simulink subsystem "DataLoader_Single_Array"  (R2019b)
settings: Solver=VariableStepAuto  StartTime=0.0  StopTime=10.0  RelTol=1e-3
settings Model: Creator=toons  LastModifiedBy=toons

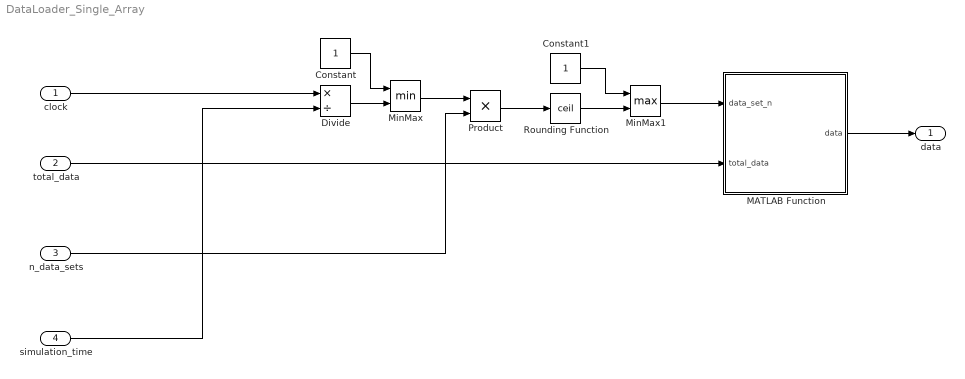
== system DataLoader_Single_Array ==
  clock : Inport
  total_data : Inport  Port=2
  n_data_sets : Inport  Port=3
  simulation_time : Inport  Port=4
  Constant : Constant
  Constant1 : Constant
  Divide : Product  Inputs=*/
  MATLAB Function : MATLAB Function  TreatAsAtomicUnit=on
  MinMax : MinMax  Inputs=2
  MinMax1 : MinMax  Function=max  Inputs=2
  Product : Product
  Rounding Function : Rounding  Operator=ceil
  data : Outport
  wires:
  clock/1 -> Divide/1
  simulation_time/1 -> Divide/2
  Divide/1 -> MinMax/2
  Constant/1 -> MinMax/1
  MinMax/1 -> Product/1
  n_data_sets/1 -> Product/2
  Product/1 -> Rounding Function/1
  total_data/1 -> MATLAB Function/2(total_data)
  MATLAB Function/1(data) -> data/1
  Rounding Function/1 -> MinMax1/2
  Constant1/1 -> MinMax1/1
  MinMax1/1 -> MATLAB Function/1(data_set_n)

== matlab function DataLoader_Single_Array/MATLAB Function ==
  data: data_set_n input; data output; total_data input
function data = squeeze_data(data_set_n, total_data)
data = squeeze(total_data(data_set_n,:,:)).';
